simulink model "uut_vdif"  (R2012b)
settings: Solver=ode45  StartTime=0.0  StopTime=sim_time  RelTol=1e-3
libraries: xbsIndex_r4 x487, casper_library_delays x9, xps_library x1
(part 1 of 4)
settings Model: Creator=lvertats  LastModifiedBy=lvertats

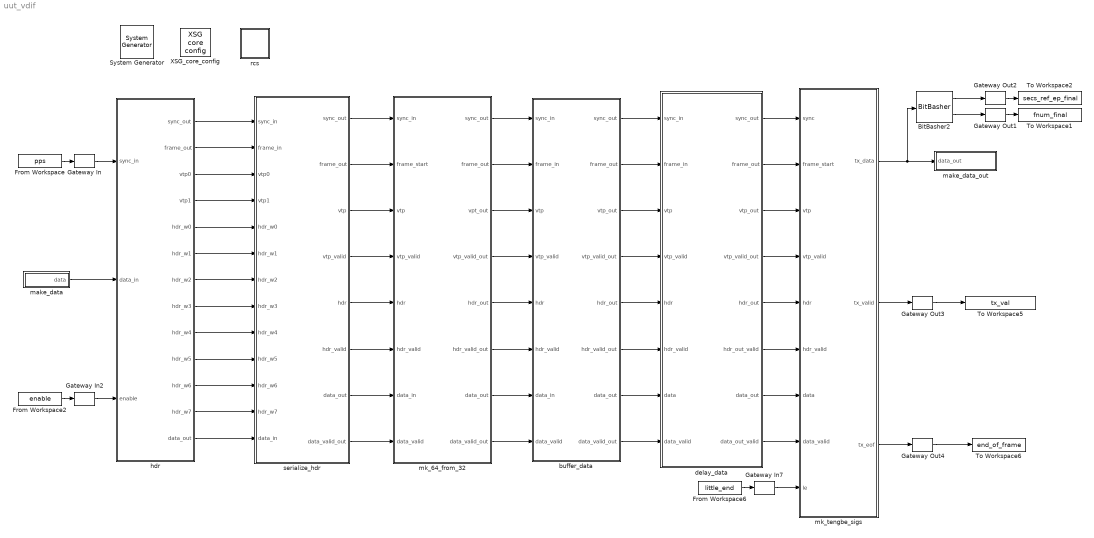
== system uut_vdif ==
  " System Generator" : xbsIndex_r4/ System Generator  Tag=genX  xilinxfamily=virtex6  part=xc6vsx475t  speed=-1  package=ff1759  synthesis_tool=XST  clock_wrapper=Clock Enables  directory=./r2dbe_top_ctr/sysgen  proj_type=Project Navigator  Synth_file=XST Defaults  Impl_file=ISE Defaults  testbench=off  simulink_period=1  sysclk_period=3.9062  dcm_input_clock_period=100  incr_netlist=off  trim_vbits=Everywhere in SubSystem  dbl_ovrd=According to Block Masks  core_generation=According to Block Masks  run_coregen=off  deprecated_control=off  eval_field=0  block_type=sysgen
      settings: block_version=11.4
  BitBasher2 : xbsIndex_r4/BitBasher  bitexpr=|  display_expr=off  sr_1=1  arith_type1=Unsigned  bin_pt1=0  sr_2=2  arith_type2=Unsigned  bin_pt2=0  sr_3=3  arith_type3=Unsigned  bin_pt3=0  sr_4=4  arith_type4="Signed  (2's comp)"  bin_pt4=0  dbl_ovrd=off  block_type=bitbasher
      | <!DOCTYPE HTML PUBLIC "-//W3C//DTD HTML 4.0//EN" "http://www.w3.org/TR/REC-html40/strict.dtd">
      | <html><head><meta name="qrichtext" content="1" /><style type="text/css">
      | p, li { white-space: pre-wrap; }
      | </style></head><body style=" font-family:'Sans'; font-size:10pt; font-weight:400; font-style:normal;">
      | <p style=" margin-top:12px; margin-bottom:12px; margin-left:0px; margin-right:0px; -qt-block-indent:0; text-indent:0px;"><span style=" font-family:'MS Shell Dlg'; font-size:8pt;">s={h[61:32]}<br />f = {h[23:0]}</span></p></body></html>
  From Workspace : FromWorkspace  VariableName=pps  Interpolate=off  OutputAfterFinalValue=Cyclic repetition
  From Workspace2 : FromWorkspace  VariableName=enable  Interpolate=off  OutputAfterFinalValue=Cyclic repetition
  From Workspace6 : FromWorkspace  VariableName=little_end  Interpolate=off  OutputAfterFinalValue=Cyclic repetition
  Gateway In : xbsIndex_r4/Gateway In  gui_display_data_type=Boolean  arith_type=Boolean  n_bits=16  bin_pt=14  preci_type=Single  exp_width=8  frac_width=24  quantization="Round  (unbiased: +/- Inf)"  overflow=Saturate  period=1  dbl_ovrd=off  timing_constraint=None  locs_specified=off  LOCs={}  UseAsADC=off  ADCChannel='1'  inherit_from_input=off  hdl_port=on  block_type=gatewayin
  Gateway In2 : xbsIndex_r4/Gateway In  gui_display_data_type=Boolean  arith_type=Boolean  n_bits=16  bin_pt=14  preci_type=Single  exp_width=8  frac_width=24  quantization="Round  (unbiased: +/- Inf)"  overflow=Saturate  period=1  dbl_ovrd=off  timing_constraint=None  locs_specified=off  LOCs={}  UseAsADC=off  ADCChannel='1'  inherit_from_input=off  hdl_port=on  block_type=gatewayin
  Gateway In7 : xbsIndex_r4/Gateway In  gui_display_data_type=Boolean  arith_type=Boolean  n_bits=16  bin_pt=14  preci_type=Single  exp_width=8  frac_width=24  quantization="Round  (unbiased: +/- Inf)"  overflow=Saturate  period=1  dbl_ovrd=off  timing_constraint=None  locs_specified=off  LOCs={}  UseAsADC=off  ADCChannel='1'  inherit_from_input=off  hdl_port=on  block_type=gatewayin
  Gateway Out{1..4} (4 alike) : xbsIndex_r4/Gateway Out  inherit_from_input=off  hdl_port=on  timing_constraint=None  locs_specified=off  LOCs={}  UseAsDAC=off  DACChannel='1'  block_type=gatewayout
  To Workspace1 : ToWorkspace  VariableName=fnum_final  SampleTime=-1  SaveFormat=Timeseries
  To Workspace2 : ToWorkspace  VariableName=secs_ref_ep_final  SampleTime=-1  SaveFormat=Timeseries
  To Workspace5 : ToWorkspace  VariableName=tx_val  SampleTime=-1  SaveFormat=Timeseries
  To Workspace6 : ToWorkspace  VariableName=end_of_frame  SampleTime=-1  SaveFormat=Timeseries
  XSG_core_config : xps_library/XSG core config  Tag=xps:xsg  hw_sys=ROACH2:sx475t  clk_src=adc0_clk  ROACH_clk_src=dac1_clk  ROACH2_clk_src=adc0_clk  MKDIG_clk_src=sys_clk  clk_rate=256.0  sample_period=1  synthesis_tool=XST
  buffer_data : Subsystem
  delay_data : Subsystem
  hdr : Subsystem
  make_data : Subsystem
  make_data_out : Subsystem
  mk_64_from_32 : Subsystem
  mk_tengbe_sigs : Subsystem
  rcs : Subsystem  AncestorBlock=casper_library_misc/rcs  mask(rcs){app_src=timestamp, lib_src=git, user_val=2704}
      mask prompts: app_src "Application revision info to capture"; lib_src "CASPER libraries revision info to capture"; user_val "User specified value"
      mask help:
      | Embeds revision control information for the user design and libraries.
      | On failure to locate specified revision information, falls back to
      | timestamps (current time for libraries).
      | A user specified value is also stored.
      mask init:
      | rcs_init(gcb, ...
      |     'app_src', app_src, ...
      |     'lib_src', lib_src);
      mask TypeOptions app_src: timestamp | git | svn
      mask TypeOptions lib_src: timestamp | git | svn
  serialize_hdr : Subsystem
  wires:
  Gateway Out2/1 -> To Workspace2/1
  BitBasher2/1 -> Gateway Out2/1
  mk_tengbe_sigs/1(tx_data) -> make_data_out/1(data_out), BitBasher2/1
  Gateway Out1/1 -> To Workspace1/1
  BitBasher2/2 -> Gateway Out1/1
  Gateway Out3/1 -> To Workspace5/1
  mk_tengbe_sigs/2(tx_valid) -> Gateway Out3/1
  Gateway Out4/1 -> To Workspace6/1
  mk_tengbe_sigs/3(tx_eof) -> Gateway Out4/1
  From Workspace6/1 -> Gateway In7/1
  delay_data/1(sync_out) -> mk_tengbe_sigs/1(sync)
  delay_data/2(frame_out) -> mk_tengbe_sigs/2(frame_start)
  delay_data/3(vtp_out) -> mk_tengbe_sigs/3(vtp)
  delay_data/4(vtp_valid_out) -> mk_tengbe_sigs/4(vtp_valid)
  delay_data/5(hdr_out) -> mk_tengbe_sigs/5(hdr)
  delay_data/6(hdr_out_valid) -> mk_tengbe_sigs/6(hdr_valid)
  delay_data/7(data_out) -> mk_tengbe_sigs/7(data)
  delay_data/8(data_out_valid) -> mk_tengbe_sigs/8(data_valid)
  Gateway In7/1 -> mk_tengbe_sigs/9(le)
  serialize_hdr/6(hdr_valid) -> mk_64_from_32/6(hdr_valid)
  serialize_hdr/3(vtp) -> mk_64_from_32/3(vtp)
  serialize_hdr/5(hdr) -> mk_64_from_32/5(hdr)
  serialize_hdr/4(vtp_valid) -> mk_64_from_32/4(vtp_valid)
  serialize_hdr/1(sync_out) -> mk_64_from_32/1(sync_in)
  serialize_hdr/2(frame_out) -> mk_64_from_32/2(frame_start)
  serialize_hdr/7(data_out) -> mk_64_from_32/7(data_in)
  mk_64_from_32/1(sync_out) -> buffer_data/1(sync_in)
  mk_64_from_32/6(hdr_valid_out) -> buffer_data/6(hdr_valid)
  mk_64_from_32/4(vtp_valid_out) -> buffer_data/4(vtp_valid)
  mk_64_from_32/5(hdr_out) -> buffer_data/5(hdr)
  mk_64_from_32/8(data_valid_out) -> buffer_data/8(data_valid)
  mk_64_from_32/3(vpt_out) -> buffer_data/3(vtp)
  mk_64_from_32/7(data_out) -> buffer_data/7(data_in)
  mk_64_from_32/2(frame_out) -> buffer_data/2(frame_in)
  serialize_hdr/8(data_valid_out) -> mk_64_from_32/8(data_valid)
  buffer_data/4(vtp_valid_out) -> delay_data/4(vtp_valid)
  buffer_data/3(vtp_out) -> delay_data/3(vtp)
  buffer_data/5(hdr_out) -> delay_data/5(hdr)
  buffer_data/2(frame_out) -> delay_data/2(frame_in)
  buffer_data/6(hdr_valid_out) -> delay_data/6(hdr_valid)
  buffer_data/1(sync_out) -> delay_data/1(sync_in)
  buffer_data/7(data_out) -> delay_data/7(data)
  buffer_data/8(data_valid_out) -> delay_data/8(data_valid)
  From Workspace/1 -> Gateway In/1
  Gateway In/1 -> hdr/1(sync_in)
  From Workspace2/1 -> Gateway In2/1
  Gateway In2/1 -> hdr/3(enable)
  make_data/1(data) -> hdr/2(data_in)
  hdr/13(data_out) -> serialize_hdr/13(" data_in")
  hdr/12(hdr_w7) -> serialize_hdr/12(" hdr_w7")
  hdr/11(hdr_w6) -> serialize_hdr/11(" hdr_w6")
  hdr/10(hdr_w5) -> serialize_hdr/10(" hdr_w5")
  hdr/9(hdr_w4) -> serialize_hdr/9(" hdr_w4")
  hdr/8(hdr_w3) -> serialize_hdr/8(" hdr_w3")
  hdr/7(hdr_w2) -> serialize_hdr/7(" hdr_w2")
  hdr/6(hdr_w1) -> serialize_hdr/6(" hdr_w1")
  hdr/5(hdr_w0) -> serialize_hdr/5(" hdr_w0")
  hdr/4(vtp1) -> serialize_hdr/4(vtp1)
  hdr/3(vtp0) -> serialize_hdr/3(vtp0)
  hdr/2(frame_out) -> serialize_hdr/2(frame_in)
  hdr/1(sync_out) -> serialize_hdr/1(sync_in)

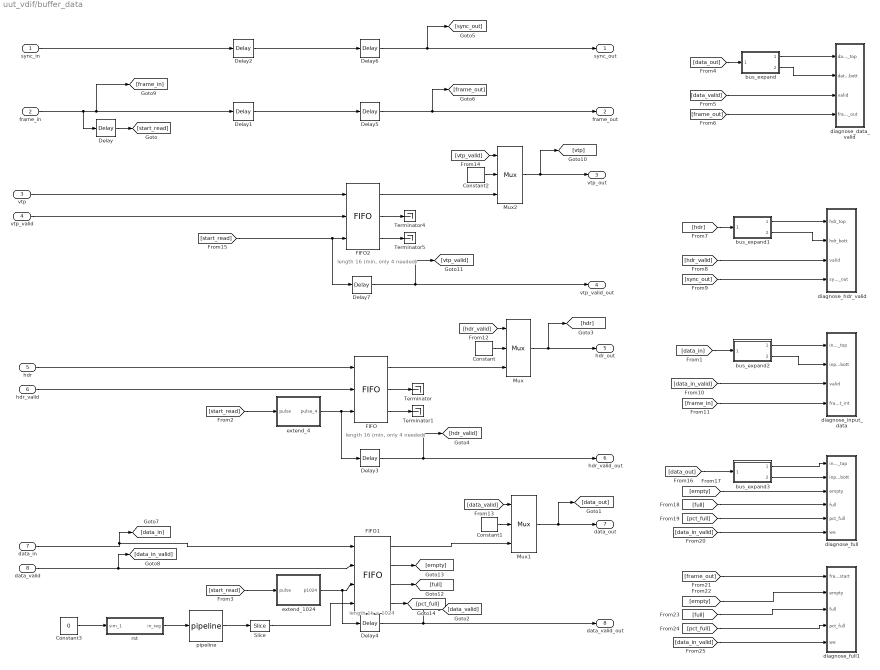
== system uut_vdif/buffer_data ==
  note: length 1k = 1024
  note: length 16 (min, only 4 needed)
  note: length 16 (min, only 4 needed)
  sync_in : Inport
  frame_in : Inport  Port=2
  vtp : Inport  Port=3
  vtp_valid : Inport  Port=4
  hdr : Inport  Port=5
  hdr_valid : Inport  Port=6
  data_in : Inport  Port=7
  data_valid : Inport  Port=8
  Constant : xbsIndex_r4/Constant  const=0  gui_display_data_type=Fixed-point  arith_type=Unsigned  n_bits=64  bin_pt=0  preci_type=Single  exp_width=8  frac_width=24  explicit_period=on  period=1  equ=P=C  opselect=C  inp2=PCIN>>17  opr=+  inp1=P  carry=CIN  dbl_ovrd=off  block_type=constant
  Constant1 : xbsIndex_r4/Constant  const=0  gui_display_data_type=Fixed-point  arith_type=Unsigned  n_bits=64  bin_pt=0  preci_type=Single  exp_width=8  frac_width=24  explicit_period=on  period=1  equ=P=C  opselect=C  inp2=PCIN>>17  opr=+  inp1=P  carry=CIN  dbl_ovrd=off  block_type=constant
  Constant2 : xbsIndex_r4/Constant  const=0  gui_display_data_type=Fixed-point  arith_type=Unsigned  n_bits=64  bin_pt=0  preci_type=Single  exp_width=8  frac_width=24  explicit_period=on  period=1  equ=P=C  opselect=C  inp2=PCIN>>17  opr=+  inp1=P  carry=CIN  dbl_ovrd=off  block_type=constant
  Constant3 : Constant  Value=0
  Delay : xbsIndex_r4/Delay  rst=off  infoeditControl=Selection of Reset will increase slice count due to use of real FFs and instead of SRLs  en=off  latency=1024  dbl_ovrd=off  reg_retiming=off  block_type=delay
  Delay1 : xbsIndex_r4/Delay  rst=off  infoeditControl=Selection of Reset will increase slice count due to use of real FFs and instead of SRLs  en=off  latency=1024  dbl_ovrd=off  reg_retiming=off  block_type=delay
  Delay2 : xbsIndex_r4/Delay  rst=off  infoeditControl=Selection of Reset will increase slice count due to use of real FFs and instead of SRLs  en=off  latency=1024  dbl_ovrd=off  reg_retiming=off  block_type=delay
  Delay{3..7} (5 alike) : xbsIndex_r4/Delay  rst=off  infoeditControl=Selection of Reset will increase slice count due to use of real FFs and instead of SRLs  en=off  latency=1  dbl_ovrd=off  reg_retiming=off  block_type=delay
  FIFO : xbsIndex_r4/FIFO  mem_type=Block RAM  performance_options=Standard_FIFO  infoedit1=Available only for V4, V5, V6, V7, K7, A7 and Zynq devices.  embedded_registers=off  depth=16  percent_nbits=1  rst=off  en=off  use_dcount=off  use_percent_full_port=off  use_almost_empty=off  almost_empty_thresh=2  use_almost_full=off  almost_full_thresh=14  dbl_ovrd=off  explicit_period=off  block_type=fifo
  FIFO1 : xbsIndex_r4/FIFO  mem_type=Block RAM  performance_options=Standard_FIFO  infoedit1=Available only for V4, V5, V6, V7, K7, A7 and Zynq devices.  embedded_registers=off  depth=1K  percent_nbits=6  rst=on  en=off  use_dcount=off  use_percent_full_port=on  use_almost_empty=off  almost_empty_thresh=2  use_almost_full=off  almost_full_thresh=14  dbl_ovrd=off  explicit_period=off  block_type=fifo
  FIFO2 : xbsIndex_r4/FIFO  mem_type=Block RAM  performance_options=Standard_FIFO  infoedit1=Available only for V4, V5, V6, V7, K7, A7 and Zynq devices.  embedded_registers=off  depth=16  percent_nbits=1  rst=off  en=off  use_dcount=off  use_percent_full_port=off  use_almost_empty=off  almost_empty_thresh=2  use_almost_full=off  almost_full_thresh=14  dbl_ovrd=off  explicit_period=off  block_type=fifo
  Mux : xbsIndex_r4/Mux  inputs=2  en=off  latency=0  precision=Full  arith_type=Unsigned  n_bits=16  bin_pt=14  quantization=Truncate  overflow=Wrap  dbl_ovrd=off  block_type=mux
  Mux1 : xbsIndex_r4/Mux  inputs=2  en=off  latency=0  precision=Full  arith_type=Unsigned  n_bits=16  bin_pt=14  quantization=Truncate  overflow=Wrap  dbl_ovrd=off  block_type=mux
  Mux2 : xbsIndex_r4/Mux  inputs=2  en=off  latency=0  precision=Full  arith_type=Unsigned  n_bits=16  bin_pt=14  quantization=Truncate  overflow=Wrap  dbl_ovrd=off  block_type=mux
  Slice : xbsIndex_r4/Slice  nbits=1  boolean_output=on  mode=Lower Bit Location + Width  bit1=0  base1=LSB of Input  bit0=0  base0=LSB of Input  dbl_ovrd=off  block_type=slice
  Terminator{,1,4..5} (4 alike) : Terminator
  bus_expand : Subsystem  AncestorBlock=casper_library_flow_control/bus_expand  mask(bus_expand){mode=divisions of equal size, outputNum=2, outputWidth=32, outputBinaryPt=0, outputArithmeticType=0, show_format=off, outputToWorkspace=off, variablePrefix=out, outputToModelAsWell=on}
      mask prompts: outputNum "Number of outputs:"; outputWidth "Output width:"; outputBinaryPt "Output binary point position:"; outputArithmeticType "Output arithmetic type (ufix=0, fix=1, bool=2):"; show_format "Print format string?"; outputToWorkspace "Output to workspace?"; variablePrefix "Variable name prefix:"; outputToModelAsWell "Output to model as well?"
      mask help:
      | Expands a 'bus' made using a bus_create or Xilinx
      | concat block.
      | The input will be divided into the specified number
      | of outputs with the specified arithmetic types.
      | Divisions are made from most significant bit.
      mask init:
      | bus_expand_init(gcb,...
      |     'mode', mode, ...
      |     'outputNum', outputNum, ...
      |     'outputWidth', outputWidth, ...
      |     'outputBinaryPt', outputBinaryPt, ...
      |     'outputArithmeticType', outputArithmeticType, ...
      |     'show_format', show_format, ...
      |     'outputToWorkspace', outputToWorkspace, ...
      |     'variablePrefix', variablePrefix, ...
      |     'outputToModelAsWell', outputToModelAsWell);
      settings: AttributesFormatString=2 outputs
      mask TypeOptions mode: divisions of equal size | divisions of arbitrary size
      mask Callback mode: bus_expand_callback();
      mask Callback outputWidth: bus_expand_callback();
      mask Callback outputToWorkspace: bus_expand_callback();
  bus_expand1 : Subsystem  AncestorBlock=casper_library_flow_control/bus_expand  mask(bus_expand){mode=divisions of equal size, outputNum=2, outputWidth=32, outputBinaryPt=0, outputArithmeticType=0, show_format=off, outputToWorkspace=off, variablePrefix=out, outputToModelAsWell=on}
      mask prompts: outputNum "Number of outputs:"; outputWidth "Output width:"; outputBinaryPt "Output binary point position:"; outputArithmeticType "Output arithmetic type (ufix=0, fix=1, bool=2):"; show_format "Print format string?"; outputToWorkspace "Output to workspace?"; variablePrefix "Variable name prefix:"; outputToModelAsWell "Output to model as well?"
      mask help:
      | Expands a 'bus' made using a bus_create or Xilinx
      | concat block.
      | The input will be divided into the specified number
      | of outputs with the specified arithmetic types.
      | Divisions are made from most significant bit.
      mask init: same as uut_vdif/buffer_data/bus_expand
      settings: AttributesFormatString=2 outputs
      mask TypeOptions mode: divisions of equal size | divisions of arbitrary size
      mask Callback mode: bus_expand_callback();
      mask Callback outputWidth: bus_expand_callback();
      mask Callback outputToWorkspace: bus_expand_callback();
  bus_expand2 : Subsystem  AncestorBlock=casper_library_flow_control/bus_expand  mask(bus_expand){mode=divisions of equal size, outputNum=2, outputWidth=32, outputBinaryPt=0, outputArithmeticType=0, show_format=off, outputToWorkspace=off, variablePrefix=out, outputToModelAsWell=on}
      mask prompts: outputNum "Number of outputs:"; outputWidth "Output width:"; outputBinaryPt "Output binary point position:"; outputArithmeticType "Output arithmetic type (ufix=0, fix=1, bool=2):"; show_format "Print format string?"; outputToWorkspace "Output to workspace?"; variablePrefix "Variable name prefix:"; outputToModelAsWell "Output to model as well?"
      mask help:
      | Expands a 'bus' made using a bus_create or Xilinx
      | concat block.
      | The input will be divided into the specified number
      | of outputs with the specified arithmetic types.
      | Divisions are made from most significant bit.
      mask init: same as uut_vdif/buffer_data/bus_expand
      settings: AttributesFormatString=2 outputs
      mask TypeOptions mode: divisions of equal size | divisions of arbitrary size
      mask Callback mode: bus_expand_callback();
      mask Callback outputWidth: bus_expand_callback();
      mask Callback outputToWorkspace: bus_expand_callback();
  bus_expand3 : Subsystem  AncestorBlock=casper_library_flow_control/bus_expand  mask(bus_expand){mode=divisions of equal size, outputNum=2, outputWidth=32, outputBinaryPt=0, outputArithmeticType=0, show_format=off, outputToWorkspace=off, variablePrefix=out, outputToModelAsWell=on}
      mask prompts: outputNum "Number of outputs:"; outputWidth "Output width:"; outputBinaryPt "Output binary point position:"; outputArithmeticType "Output arithmetic type (ufix=0, fix=1, bool=2):"; show_format "Print format string?"; outputToWorkspace "Output to workspace?"; variablePrefix "Variable name prefix:"; outputToModelAsWell "Output to model as well?"
      mask help:
      | Expands a 'bus' made using a bus_create or Xilinx
      | concat block.
      | The input will be divided into the specified number
      | of outputs with the specified arithmetic types.
      | Divisions are made from most significant bit.
      mask init: same as uut_vdif/buffer_data/bus_expand
      settings: AttributesFormatString=2 outputs
      mask TypeOptions mode: divisions of equal size | divisions of arbitrary size
      mask Callback mode: bus_expand_callback();
      mask Callback outputWidth: bus_expand_callback();
      mask Callback outputToWorkspace: bus_expand_callback();
  diagnose_data_valid : Subsystem
  diagnose_full : Subsystem
  diagnose_full1 : Subsystem
  diagnose_hdr_valid : Subsystem
  diagnose_input_data : Subsystem
  extend_1024 : Subsystem
  extend_4 : Subsystem
  pipeline : casper_library_delays/pipeline  latency=3
      settings: AttributesFormatString=Latency = %<latency>
  rst : Subsystem  Tag=xps:sw_reg  AncestorBlock=xps_library/software register  mask(swreg){mode=one value, io_dir=From Processor, io_delay=0, sample_period=1, names=reg, bitwidths=32, arith_types=0, bin_pts=0, sim_port=on, show_format=off}
      mask prompts: io_dir "I/O direction"; io_delay "I/O delay"; sample_period "Sample period"; names "Name:"; bitwidths "Bitwidth:"; arith_types "Type (ufix=0, fix=1, bool=2):"; bin_pts "Binary pt:"; sim_port "Provide sim input/output?"; show_format "Print format string?"
      mask init:
      | swreg_init(gcb)
      settings: AttributesFormatString=1input
      mask TypeOptions mode: one value | fields of equal size | fields of arbitrary size
      mask Callback mode: swreg_cb(gcb);
      mask TypeOptions io_dir: To Processor | From Processor
      mask Callback io_dir:
      | mask_enables = get_param(gcb, 'MaskEnables');
      | mask_names = get_param(gcb, 'MaskNames');
      | if strcmp(get_param(gcb, 'io_dir'), 'To Processor'),
      |     mask_enables{ismember(mask_names, 'sample_period')} = 'off';
      | else
      |     mask_enables{ismember(mask_names, 'sample_period')} = 'on';
      | end
      | set_param(gcb, 'MaskEnables', mask_enables);
      mask Callback bitwidths:
      | swreg_maskcheck(gcb);
      | % blk = gcb;
      | % mode = get_param(blk, 'mode');
      | % current_widths = eval(get_param(blk, 'bitwidths'));
      | % if (strcmp(mode, 'one value') || strcmp(mode, 'fields of equal size')) && (length(current_widths) > 1),
      | %     error('Only one width may be specified for this mode.');
      | % elseif strcmp(mode, 'fields of arbitrary size')
      | %     current_names = textscan(strtrim(strrep(strrep(get_param(blk, 'names'), ']', ''), '[', '')), '%s');
      | %     current_names = current_names{1};
      | %     numios = length(current_names);
      | %     if length(current_widths) ~= numios,
      | %         error('%d field names specified, but %d widths?', numios, length(current_widths));
      | %     end
      | % end
      | % total_width = 0;
      | % for ctr = 1 : length(current_widths),
      | %     total_width = total_width + current_widths(ctr);
      | % end
      | % if total_width > 32,
      | %     error('Total width must be 32 or less, set to %d.', total_width);
      | % end
      mask Callback arith_types:
      | [numios, ~, ~, ~, current_types] = swreg_maskcheck(gcb);
      | % blk = gcb;
      | % mode = get_param(blk, 'mode');
      | % current_types = eval(get_param(blk, 'arith_types'));
      | % numios = length(current_types);
      | % if (strcmp(mode, 'one value') || strcmp(mode, 'fields of equal size')) && (length(current_types) > 1),
      | %     error('Only one type may be specified for this mode.');
      | % elseif strcmp(mode, 'fields of arbitrary size')
      | %     current_names = textscan(strtrim(strrep(strrep(get_param(blk, 'names'), ']', ''), '[', '')), '%s');
      | %     current_names = current_names{1};
      | %     numios = length(current_names);
      | %     if length(current_types) ~= numios,
      | %         error('%d field names specified, but %d types?', numios, length(current_types));
      | %     end
      | % end
      | problem = 0;
      | for ctr = 1 : numios,
      |     t = current_types(ctr);
      |     if (t < 0) || (t > 2),
      |         problem = t;
      |         ctr = numios + 1;
      |     end
      | end
      | if problem ~= 0,
      |     error('Type cannot be %i, must be 0, 1 or 2.', problem);
      | end
      mask Callback bin_pts:
      | swreg_maskcheck(gcb);
      | % blk = gcb;
      | % mode = get_param(blk, 'mode');
      | % current_bins = eval(get_param(blk, 'bin_pts'));
      | % if (strcmp(mode, 'one value') || strcmp(mode, 'fields of equal size')) && (length(current_bins) > 1),
      | %     error('Only one binary pt may be specified for this mode.');
      | % elseif strcmp(mode, 'fields of arbitrary size')
      | %     current_names = textscan(strtrim(strrep(strrep(get_param(blk, 'names'), ']', ''), '[', '')), '%s');
      | %     current_names = current_names{1};
      | %     numios = length(current_names);
      | %     if length(current_bins) ~= numios,
      | %         error('%d field names specified, but %d binary pts?', numios, length(current_bins));
      | %     end
      | % end
  sync_out : Outport
  frame_out : Outport  Port=2
  vtp_out : Outport  Port=3
  vtp_valid_out : Outport  Port=4
  hdr_out : Outport  Port=5
  hdr_valid_out : Outport  Port=6
  data_out : Outport  Port=7
  data_valid_out : Outport  Port=8
  wires:
  sync_in/1 -> Delay2/1
  Delay/1 -> [start_read]
  hdr/1 -> FIFO/1
  hdr_valid/1 -> FIFO/2
  [start_read] -> extend_4/1(pulse)
  extend_4/1(pulse_4) -> Delay3/1, FIFO/3
  FIFO/1 -> Mux/3
  data_in/1 -> [data_in], FIFO1/1
  data_valid/1 -> [data_in_valid], FIFO1/2
  [start_read] -> extend_1024/1(pulse)
  extend_1024/1(p1024) -> Delay4/1, FIFO1/3
  FIFO1/1 -> Mux1/3
  FIFO/2 -> Terminator/1
  FIFO/3 -> Terminator1/1
  FIFO1/2 -> [empty]
  FIFO1/3 -> [full]
  bus_expand/2(lsb_out1) -> diagnose_data_valid/2(data_bott)
  bus_expand/1(msb_out2) -> diagnose_data_valid/1(data_top)
  [data_valid] -> diagnose_data_valid/3(valid)
  [frame_out] -> diagnose_data_valid/4(frame_start_out)
  [data_out] -> bus_expand/1(bus_in)
  frame_in/1 -> Delay/1, [frame_in], Delay1/1
  bus_expand1/2(lsb_out1) -> diagnose_hdr_valid/2(hdr_bott)
  bus_expand1/1(msb_out2) -> diagnose_hdr_valid/1(hdr_top)
  [hdr_valid] -> diagnose_hdr_valid/3(valid)
  [sync_out] -> diagnose_hdr_valid/4(sync_out)
  [hdr] -> bus_expand1/1(bus_in)
  Delay1/1 -> Delay5/1
  Delay2/1 -> Delay6/1
  bus_expand2/2(lsb_out1) -> diagnose_input_data/2(input_data_bott)
  bus_expand2/1(msb_out2) -> diagnose_input_data/1(input_data_top)
  [data_in_valid] -> diagnose_input_data/3(valid)
  [frame_in] -> diagnose_input_data/4(frame_start_int)
  [data_in] -> bus_expand2/1(bus_in)
  Delay3/1 -> hdr_valid_out/1, [hdr_valid]
  Delay4/1 -> data_valid_out/1, [data_valid]
  Delay5/1 -> frame_out/1, [frame_out]
  Delay6/1 -> [sync_out], sync_out/1
  Constant/1 -> Mux/2
  Mux/1 -> hdr_out/1, [hdr]
  [hdr_valid] -> Mux/1
  Constant1/1 -> Mux1/2
  [data_valid] -> Mux1/1
  Mux1/1 -> data_out/1, [data_out]
  vtp/1 -> FIFO2/1
  vtp_valid/1 -> FIFO2/2
  [start_read] -> FIFO2/3, Delay7/1
  FIFO2/1 -> Mux2/3
  FIFO2/2 -> Terminator4/1
  FIFO2/3 -> Terminator5/1
  Delay7/1 -> vtp_valid_out/1, [vtp_valid]
  Constant2/1 -> Mux2/2
  Mux2/1 -> vtp_out/1, [vtp]
  [vtp_valid] -> Mux2/1
  bus_expand3/2(lsb_out1) -> diagnose_full/2(input_data_bott)
  bus_expand3/1(msb_out2) -> diagnose_full/1(input_data_top)
  [empty] -> diagnose_full/3(empty)
  [full] -> diagnose_full/4(full)
  [data_out] -> bus_expand3/1(bus_in)
  [pct_full] -> diagnose_full/5(pct_full)
  [data_in_valid] -> diagnose_full/6(we)
  FIFO1/4 -> [pct_full]
  [empty] -> diagnose_full1/2(empty)
  [full] -> diagnose_full1/3(full)
  [pct_full] -> diagnose_full1/4(pct_full)
  [data_in_valid] -> diagnose_full1/5(we)
  [frame_out] -> diagnose_full1/1(frame_start)
  rst/1(in_reg) -> pipeline/1
  pipeline/1 -> Slice/1
  Constant3/1 -> rst/1(sim_1)
  Slice/1 -> FIFO1/4

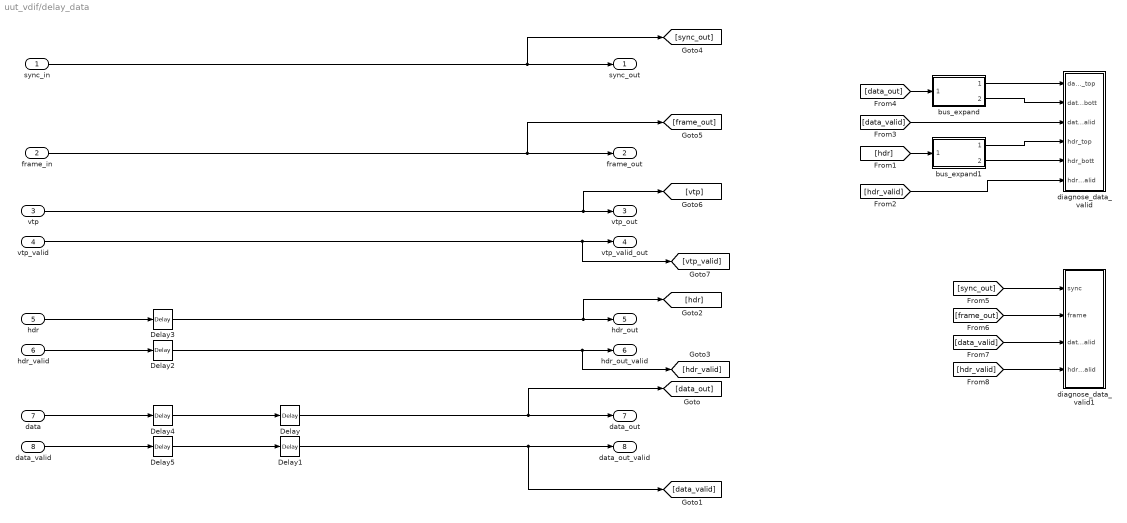
== system uut_vdif/delay_data ==
  sync_in : Inport
  frame_in : Inport  Port=2
  vtp : Inport  Port=3
  vtp_valid : Inport  Port=4
  hdr : Inport  Port=5
  hdr_valid : Inport  Port=6
  data : Inport  Port=7
  data_valid : Inport  Port=8
  Delay : xbsIndex_r4/Delay  rst=off  infoeditControl=Selection of Reset will increase slice count due to use of real FFs and instead of SRLs  en=off  latency=4  dbl_ovrd=off  reg_retiming=off  block_type=delay
  Delay1 : xbsIndex_r4/Delay  rst=off  infoeditControl=Selection of Reset will increase slice count due to use of real FFs and instead of SRLs  en=off  latency=4  dbl_ovrd=off  reg_retiming=off  block_type=delay
  Delay{2..5} (4 alike) : xbsIndex_r4/Delay  rst=off  infoeditControl=Selection of Reset will increase slice count due to use of real FFs and instead of SRLs  en=off  latency=1  dbl_ovrd=off  reg_retiming=off  block_type=delay
  bus_expand : Subsystem  AncestorBlock=casper_library_flow_control/bus_expand  mask(bus_expand){mode=divisions of equal size, outputNum=2, outputWidth=32, outputBinaryPt=0, outputArithmeticType=0, show_format=off, outputToWorkspace=off, variablePrefix=out, outputToModelAsWell=on}
      mask prompts: outputNum "Number of outputs:"; outputWidth "Output width:"; outputBinaryPt "Output binary point position:"; outputArithmeticType "Output arithmetic type (ufix=0, fix=1, bool=2):"; show_format "Print format string?"; outputToWorkspace "Output to workspace?"; variablePrefix "Variable name prefix:"; outputToModelAsWell "Output to model as well?"
      mask help:
      | Expands a 'bus' made using a bus_create or Xilinx
      | concat block.
      | The input will be divided into the specified number
      | of outputs with the specified arithmetic types.
      | Divisions are made from most significant bit.
      mask init: same as uut_vdif/buffer_data/bus_expand
      settings: AttributesFormatString=2 outputs
      mask TypeOptions mode: divisions of equal size | divisions of arbitrary size
      mask Callback mode: bus_expand_callback();
      mask Callback outputWidth: bus_expand_callback();
      mask Callback outputToWorkspace: bus_expand_callback();
  bus_expand1 : Subsystem  AncestorBlock=casper_library_flow_control/bus_expand  mask(bus_expand){mode=divisions of equal size, outputNum=2, outputWidth=32, outputBinaryPt=0, outputArithmeticType=0, show_format=off, outputToWorkspace=off, variablePrefix=out, outputToModelAsWell=on}
      mask prompts: outputNum "Number of outputs:"; outputWidth "Output width:"; outputBinaryPt "Output binary point position:"; outputArithmeticType "Output arithmetic type (ufix=0, fix=1, bool=2):"; show_format "Print format string?"; outputToWorkspace "Output to workspace?"; variablePrefix "Variable name prefix:"; outputToModelAsWell "Output to model as well?"
      mask help:
      | Expands a 'bus' made using a bus_create or Xilinx
      | concat block.
      | The input will be divided into the specified number
      | of outputs with the specified arithmetic types.
      | Divisions are made from most significant bit.
      mask init: same as uut_vdif/buffer_data/bus_expand
      settings: AttributesFormatString=2 outputs
      mask TypeOptions mode: divisions of equal size | divisions of arbitrary size
      mask Callback mode: bus_expand_callback();
      mask Callback outputWidth: bus_expand_callback();
      mask Callback outputToWorkspace: bus_expand_callback();
  diagnose_data_valid : Subsystem
  diagnose_data_valid1 : Subsystem
  sync_out : Outport
  frame_out : Outport  Port=2
  vtp_out : Outport  Port=3
  vtp_valid_out : Outport  Port=4
  hdr_out : Outport  Port=5
  hdr_out_valid : Outport  Port=6
  data_out : Outport  Port=7
  data_out_valid : Outport  Port=8
  wires:
  [data_out] -> bus_expand/1(bus_in)
  bus_expand/1(msb_out2) -> diagnose_data_valid/1(data_top)
  bus_expand/2(lsb_out1) -> diagnose_data_valid/2(data_bott)
  sync_in/1 -> [sync_out], sync_out/1
  frame_in/1 -> [frame_out], frame_out/1
  hdr/1 -> Delay3/1
  hdr_valid/1 -> Delay2/1
  data/1 -> Delay4/1
  Delay/1 -> [data_out], data_out/1
  data_valid/1 -> Delay5/1
  Delay1/1 -> [data_valid], data_out_valid/1
  [hdr] -> bus_expand1/1(bus_in)
  bus_expand1/1(msb_out2) -> diagnose_data_valid/4(hdr_top)
  bus_expand1/2(lsb_out1) -> diagnose_data_valid/5(hdr_bott)
  [data_valid] -> diagnose_data_valid/3(data_valid)
  [hdr_valid] -> diagnose_data_valid/6(hdr_valid)
  [sync_out] -> diagnose_data_valid1/1(sync)
  [frame_out] -> diagnose_data_valid1/2(frame)
  [data_valid] -> diagnose_data_valid1/3(data_valid)
  [hdr_valid] -> diagnose_data_valid1/4(hdr_valid)
  vtp/1 -> vtp_out/1, [vtp]
  vtp_valid/1 -> vtp_valid_out/1, [vtp_valid]
  Delay2/1 -> [hdr_valid], hdr_out_valid/1
  Delay3/1 -> [hdr], hdr_out/1
  Delay4/1 -> Delay/1
  Delay5/1 -> Delay1/1

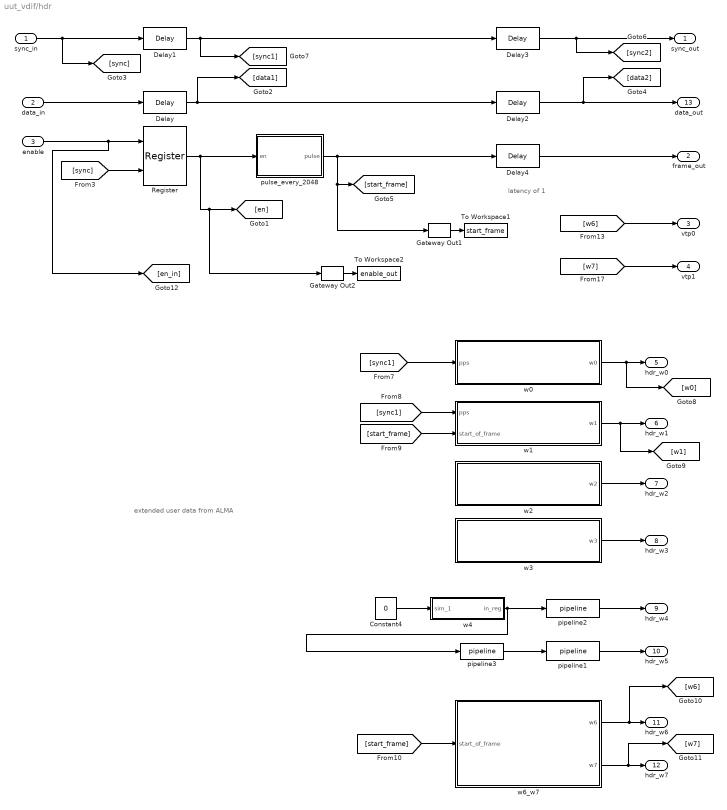
== system uut_vdif/hdr ==
  note: latency of 1
  note: extended user data
      | from ALMA
  sync_in : Inport
  data_in : Inport  Port=2
  enable : Inport  Port=3
  Constant4 : Constant  Value=0
  Delay{,1..4} (5 alike) : xbsIndex_r4/Delay  rst=off  infoeditControl=Selection of Reset will increase slice count due to use of real FFs and instead of SRLs  en=off  latency=1  dbl_ovrd=off  reg_retiming=off  block_type=delay
  Gateway Out1 : xbsIndex_r4/Gateway Out  inherit_from_input=off  hdl_port=on  timing_constraint=None  locs_specified=off  LOCs={}  UseAsDAC=off  DACChannel='1'  block_type=gatewayout
  Gateway Out2 : xbsIndex_r4/Gateway Out  inherit_from_input=off  hdl_port=on  timing_constraint=None  locs_specified=off  LOCs={}  UseAsDAC=off  DACChannel='1'  block_type=gatewayout
  Register : xbsIndex_r4/Register  init=0  rst=off  en=on  dbl_ovrd=off  block_type=register
  To Workspace1 : ToWorkspace  VariableName=start_frame  SampleTime=-1  SaveFormat=Timeseries
  To Workspace2 : ToWorkspace  VariableName=enable_out  SampleTime=-1  SaveFormat=Timeseries
  pipeline1 : casper_library_delays/pipeline  latency=1
      settings: AttributesFormatString=Latency = %<latency>
  pipeline2 : casper_library_delays/pipeline  latency=1
      settings: AttributesFormatString=Latency = %<latency>
  pipeline3 : casper_library_delays/pipeline  latency=3
      settings: AttributesFormatString=Latency = %<latency>
  pulse_every_2048 : Subsystem  mask{per=2048}
      mask prompts: per "period"
      mask help: Creates a pulse duration 1 with period from 2 to <large number>. Pulse begins with enable signal, no latency.
  w0 : Subsystem
  w1 : Subsystem
  w2 : Subsystem
  w3 : Subsystem
  w4 : Subsystem  Tag=xps:sw_reg  AncestorBlock=xps_library/software register  mask(swreg){mode=one value, io_dir=From Processor, io_delay=0, sample_period=1, names=reg, bitwidths=32, arith_types=0, bin_pts=0, sim_port=on, show_format=off}
      mask prompts: io_dir "I/O direction"; io_delay "I/O delay"; sample_period "Sample period"; names "Name:"; bitwidths "Bitwidth:"; arith_types "Type (ufix=0, fix=1, bool=2):"; bin_pts "Binary pt:"; sim_port "Provide sim input/output?"; show_format "Print format string?"
      mask init:
      | swreg_init(gcb)
      settings: AttributesFormatString=1input
      mask TypeOptions mode: one value | fields of equal size | fields of arbitrary size
      mask Callback mode: swreg_cb(gcb);
      mask TypeOptions io_dir: To Processor | From Processor
      mask Callback io_dir:
      | mask_enables = get_param(gcb, 'MaskEnables');
      | mask_names = get_param(gcb, 'MaskNames');
      | if strcmp(get_param(gcb, 'io_dir'), 'To Processor'),
      |     mask_enables{ismember(mask_names, 'sample_period')} = 'off';
      | else
      |     mask_enables{ismember(mask_names, 'sample_period')} = 'on';
      | end
      | set_param(gcb, 'MaskEnables', mask_enables);
      mask Callback bitwidths:
      | swreg_maskcheck(gcb);
      | % blk = gcb;
      | % mode = get_param(blk, 'mode');
      | % current_widths = eval(get_param(blk, 'bitwidths'));
      | % if (strcmp(mode, 'one value') || strcmp(mode, 'fields of equal size')) && (length(current_widths) > 1),
      | %     error('Only one width may be specified for this mode.');
      | % elseif strcmp(mode, 'fields of arbitrary size')
      | %     current_names = textscan(strtrim(strrep(strrep(get_param(blk, 'names'), ']', ''), '[', '')), '%s');
      | %     current_names = current_names{1};
      | %     numios = length(current_names);
      | %     if length(current_widths) ~= numios,
      | %         error('%d field names specified, but %d widths?', numios, length(current_widths));
      | %     end
      | % end
      | % total_width = 0;
      | % for ctr = 1 : length(current_widths),
      | %     total_width = total_width + current_widths(ctr);
      | % end
      | % if total_width > 32,
      | %     error('Total width must be 32 or less, set to %d.', total_width);
      | % end
      mask Callback arith_types:
      | [numios, ~, ~, ~, current_types] = swreg_maskcheck(gcb);
      | % blk = gcb;
      | % mode = get_param(blk, 'mode');
      | % current_types = eval(get_param(blk, 'arith_types'));
      | % numios = length(current_types);
      | % if (strcmp(mode, 'one value') || strcmp(mode, 'fields of equal size')) && (length(current_types) > 1),
      | %     error('Only one type may be specified for this mode.');
      | % elseif strcmp(mode, 'fields of arbitrary size')
      | %     current_names = textscan(strtrim(strrep(strrep(get_param(blk, 'names'), ']', ''), '[', '')), '%s');
      | %     current_names = current_names{1};
      | %     numios = length(current_names);
      | %     if length(current_types) ~= numios,
      | %         error('%d field names specified, but %d types?', numios, length(current_types));
      | %     end
      | % end
      | problem = 0;
      | for ctr = 1 : numios,
      |     t = current_types(ctr);
      |     if (t < 0) || (t > 2),
      |         problem = t;
      |         ctr = numios + 1;
      |     end
      | end
      | if problem ~= 0,
      |     error('Type cannot be %i, must be 0, 1 or 2.', problem);
      | end
      mask Callback bin_pts:
      | swreg_maskcheck(gcb);
      | % blk = gcb;
      | % mode = get_param(blk, 'mode');
      | % current_bins = eval(get_param(blk, 'bin_pts'));
      | % if (strcmp(mode, 'one value') || strcmp(mode, 'fields of equal size')) && (length(current_bins) > 1),
      | %     error('Only one binary pt may be specified for this mode.');
      | % elseif strcmp(mode, 'fields of arbitrary size')
      | %     current_names = textscan(strtrim(strrep(strrep(get_param(blk, 'names'), ']', ''), '[', '')), '%s');
      | %     current_names = current_names{1};
      | %     numios = length(current_names);
      | %     if length(current_bins) ~= numios,
      | %         error('%d field names specified, but %d binary pts?', numios, length(current_bins));
      | %     end
      | % end
  w6_w7 : Subsystem
  sync_out : Outport
  frame_out : Outport  Port=2
  vtp0 : Outport  Port=3
  vtp1 : Outport  Port=4
  hdr_w0 : Outport  Port=5
  hdr_w1 : Outport  Port=6
  hdr_w2 : Outport  Port=7
  hdr_w3 : Outport  Port=8
  hdr_w4 : Outport  Port=9
  hdr_w5 : Outport  Port=10
  hdr_w6 : Outport  Port=11
  hdr_w7 : Outport  Port=12
  data_out : Outport  Port=13
  wires:
  w4/1(in_reg) -> pipeline2/1, pipeline3/1
  Constant4/1 -> w4/1(sim_1)
  [start_frame] -> w1/2(start_of_frame)
  [sync1] -> w1/1(pps)
  [sync1] -> w0/1(pps)
  sync_in/1 -> [sync], Delay1/1
  data_in/1 -> Delay/1
  w0/1(w0) -> hdr_w0/1, [w0]
  w1/1(w1) -> hdr_w1/1, [w1]
  w2/1(w2) -> hdr_w2/1
  w3/1(w3) -> hdr_w3/1
  pipeline2/1 -> hdr_w4/1
  pipeline1/1 -> hdr_w5/1
  w6_w7/1(w6) -> hdr_w6/1, [w6]
  w6_w7/2(w7) -> hdr_w7/1, [w7]
  [start_frame] -> w6_w7/1(start_of_frame)
  pulse_every_2048/1(pulse) -> Delay4/1, [start_frame], Gateway Out1/1
  enable/1 -> [en_in], Register/1
  [sync] -> Register/2
  Delay/1 -> [data1], Delay2/1
  Delay1/1 -> Delay3/1, [sync1]
  Delay2/1 -> data_out/1, [data2]
  Delay3/1 -> [sync2], sync_out/1
  Delay4/1 -> frame_out/1
  [w6] -> vtp0/1
  [w7] -> vtp1/1
  pipeline3/1 -> pipeline1/1
  Gateway Out1/1 -> To Workspace1/1
  Register/1 -> Gateway Out2/1, [en], pulse_every_2048/1(en)
  Gateway Out2/1 -> To Workspace2/1

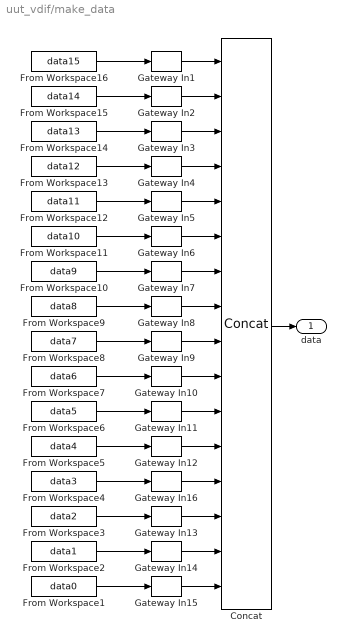
== system uut_vdif/make_data ==
  Concat : xbsIndex_r4/Concat  num_inputs=16  dbl_ovrd=off  block_type=concat
  From Workspace1 : FromWorkspace  VariableName=data0  Interpolate=off  OutputAfterFinalValue=Cyclic repetition
  From Workspace10 : FromWorkspace  VariableName=data9  Interpolate=off  OutputAfterFinalValue=Cyclic repetition
  From Workspace11 : FromWorkspace  VariableName=data10  Interpolate=off  OutputAfterFinalValue=Cyclic repetition
  From Workspace12 : FromWorkspace  VariableName=data11  Interpolate=off  OutputAfterFinalValue=Cyclic repetition
  From Workspace13 : FromWorkspace  VariableName=data12  Interpolate=off  OutputAfterFinalValue=Cyclic repetition
  From Workspace14 : FromWorkspace  VariableName=data13  Interpolate=off  OutputAfterFinalValue=Cyclic repetition
  From Workspace15 : FromWorkspace  VariableName=data14  Interpolate=off  OutputAfterFinalValue=Cyclic repetition
  From Workspace16 : FromWorkspace  VariableName=data15  Interpolate=off  OutputAfterFinalValue=Cyclic repetition
  From Workspace2 : FromWorkspace  VariableName=data1  Interpolate=off  OutputAfterFinalValue=Cyclic repetition
  From Workspace3 : FromWorkspace  VariableName=data2  Interpolate=off  OutputAfterFinalValue=Cyclic repetition
  From Workspace4 : FromWorkspace  VariableName=data3  Interpolate=off  OutputAfterFinalValue=Cyclic repetition
  From Workspace5 : FromWorkspace  VariableName=data4  Interpolate=off  OutputAfterFinalValue=Cyclic repetition
  From Workspace6 : FromWorkspace  VariableName=data5  Interpolate=off  OutputAfterFinalValue=Cyclic repetition
  From Workspace7 : FromWorkspace  VariableName=data6  Interpolate=off  OutputAfterFinalValue=Cyclic repetition
  From Workspace8 : FromWorkspace  VariableName=data7  Interpolate=off  OutputAfterFinalValue=Cyclic repetition
  From Workspace9 : FromWorkspace  VariableName=data8  Interpolate=off  OutputAfterFinalValue=Cyclic repetition
  Gateway In{1..16} (16 alike) : xbsIndex_r4/Gateway In  gui_display_data_type=Fixed-point  arith_type=Unsigned  n_bits=2  bin_pt=0  preci_type=Single  exp_width=8  frac_width=24  quantization="Round  (unbiased: +/- Inf)"  overflow=Saturate  period=1  dbl_ovrd=off  timing_constraint=None  locs_specified=off  LOCs={}  UseAsADC=off  ADCChannel='1'  inherit_from_input=off  hdl_port=on  block_type=gatewayin
  data : Outport
  wires:
  Concat/1 -> data/1
  Gateway In1/1 -> Concat/1
  Gateway In3/1 -> Concat/3
  Gateway In2/1 -> Concat/2
  Gateway In5/1 -> Concat/5
  Gateway In6/1 -> Concat/6
  Gateway In7/1 -> Concat/7
  Gateway In8/1 -> Concat/8
  Gateway In9/1 -> Concat/9
  Gateway In10/1 -> Concat/10
  Gateway In11/1 -> Concat/11
  Gateway In12/1 -> Concat/12
  Gateway In16/1 -> Concat/13
  Gateway In13/1 -> Concat/14
  Gateway In14/1 -> Concat/15
  Gateway In15/1 -> Concat/16
  Gateway In4/1 -> Concat/4
  From Workspace16/1 -> Gateway In1/1
  From Workspace15/1 -> Gateway In2/1
  From Workspace14/1 -> Gateway In3/1
  From Workspace13/1 -> Gateway In4/1
  From Workspace12/1 -> Gateway In5/1
  From Workspace11/1 -> Gateway In6/1
  From Workspace10/1 -> Gateway In7/1
  From Workspace9/1 -> Gateway In8/1
  From Workspace8/1 -> Gateway In9/1
  From Workspace7/1 -> Gateway In10/1
  From Workspace6/1 -> Gateway In11/1
  From Workspace5/1 -> Gateway In12/1
  From Workspace4/1 -> Gateway In16/1
  From Workspace3/1 -> Gateway In13/1
  From Workspace2/1 -> Gateway In14/1
  From Workspace1/1 -> Gateway In15/1
